simulink model "Ps3"  (R2020b)
settings: Solver=VariableStepAuto  StartTime=0.0  StopTime=10  RelTol=1e-3
values from neighbouring files (symbols this model uses):
  b = 50    [ps3.m]
  m = 1000    [ps3.m]
settings Model: DataDictionary=Dd.sldd  OrderedModelArguments=off  Creator=prana  LastModifiedBy=prana

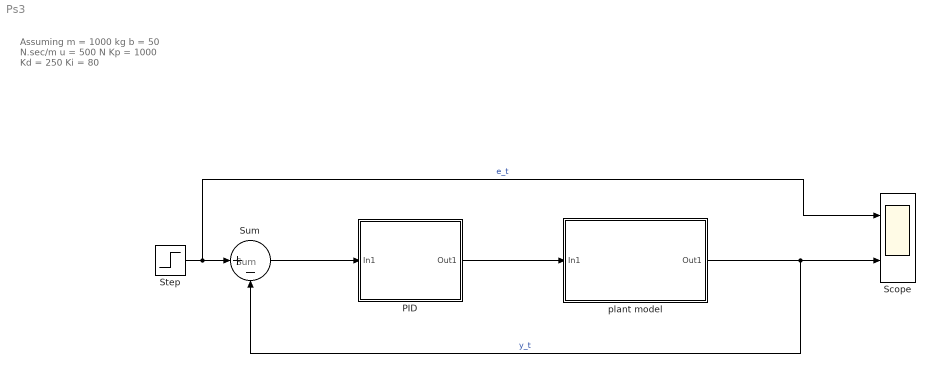
== system Ps3 ==
  note: Assuming
      | m = 1000 kg
      | b = 50 N.sec/m
      | u = 500 N
      | Kp = 1000
      | Kd = 250
      | Ki = 80
  note: Sum
  PID : Subsystem
  Scope : Scope  NumInputPorts=2
  Step : Step  Time=0  After=u  SampleTime=0
  Sum : Sum  Inputs=|+-
  plant model : Subsystem
  wires:
  Step/1 -> Scope/1, Sum/1  "e_t"
  plant model/1(Out1) -> Sum/2, Scope/2  "y_t"
  Sum/1 -> PID/1(In1)
  PID/1(Out1) -> plant model/1(In1)

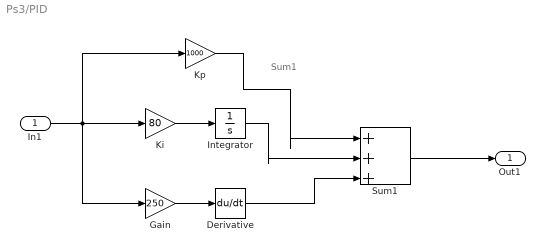
== system Ps3/PID ==
  note: Sum1
  In1 : Inport
  Derivative : Derivative
  Gain : Gain  Gain=250
  Integrator : Integrator
  Ki : Gain  Gain=80
  Kp : Gain  Gain=1000
  Sum1 : Sum  Inputs=|+++
  Out1 : Outport
  wires:
  Kp/1 -> Sum1/1
  In1/1 -> Gain/1, Ki/1, Kp/1
  Ki/1 -> Integrator/1
  Sum1/1 -> Out1/1
  Integrator/1 -> Sum1/2
  Gain/1 -> Derivative/1
  Derivative/1 -> Sum1/3

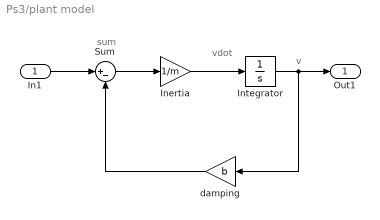
== system Ps3/plant model ==
  note: vdot
  note: sum
  note: v
  In1 : Inport
  Inertia : Gain  Gain=1/m
  Integrator : Integrator
  Sum : Sum  Inputs=|+-
  damping : Gain  Gain=b
  Out1 : Outport
  wires:
  In1/1 -> Sum/1
  Sum/1 -> Inertia/1
  Inertia/1 -> Integrator/1
  damping/1 -> Sum/2
  Integrator/1 -> Out1/1, damping/1
